simulink model "line_buffer_11x11"  (R2015a)
settings: Solver=ode45  StartTime=0.0  StopTime=10.0  RelTol=1e-3
InitFcn:
  | %% DSPBuilder Start
  | alt_dspbuilder_update_model(bdroot)
  | %% DSPBuilder End
libraries: allblocks_alteradspbuilder2 x11
settings Model: Creator=ASUS  LastModifiedBy=ASUS

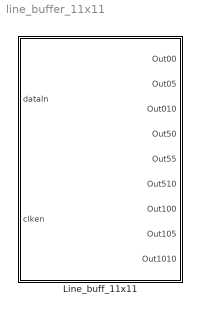
== system line_buffer_11x11 ==
  Line_buff_11x11 : Subsystem

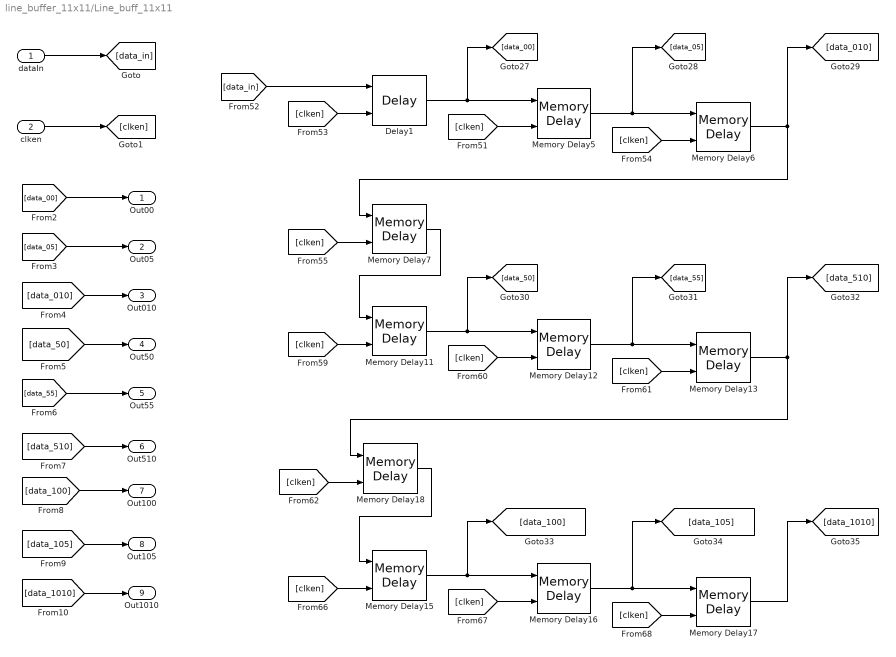
== system line_buffer_11x11/Line_buff_11x11 ==
  dataIn : Inport
  clken : Inport  Port=2
  Delay1 : allblocks_alteradspbuilder2/Delay  pipeline=1  pipeline_display=1  ClockPhase=1  use_ena=on  use_sclr=off  allowFloatingPointOverride=on  logOutputs=off  logFile=C:\Users\ASUS\Desktop\sift_fpga_final\Octave_1\line_buffer\tb_line_buffer_15x15\line%5Fbuffer%5F15x15_Line%5Fbuff%5F11x11_Delay1.fixedpointlog  use_init=off  reset_value=1
  Memory Delay11 : allblocks_alteradspbuilder2/Memory Delay  BusType=Unsigned Integer  bwl=8  bwr=0  pipeline=630  pipeline_display=630  ram_type=AUTO  use_ena=on  use_sclr=off  allowFloatingPointOverride=on  logOutputs=off  logFile=C:\Users\ASUS\Desktop\sift_fpga_final\Octave_1\line_buffer\tb_line_buffer_15x15\line%5Fbuffer%5F15x15_Line%5Fbuff%5F11x11_Memory+Delay11.fixedpointlog
  Memory Delay12 : allblocks_alteradspbuilder2/Memory Delay  BusType=Unsigned Integer  bwl=8  bwr=0  pipeline=5  pipeline_display=5  ram_type=AUTO  use_ena=on  use_sclr=off  allowFloatingPointOverride=on  logOutputs=off  logFile=C:\Users\ASUS\Desktop\sift_fpga_final\Octave_1\line_buffer\tb_line_buffer_15x15\line%5Fbuffer%5F15x15_Line%5Fbuff%5F11x11_Memory+Delay12.fixedpointlog
  Memory Delay13 : allblocks_alteradspbuilder2/Memory Delay  BusType=Unsigned Integer  bwl=8  bwr=0  pipeline=5  pipeline_display=5  ram_type=AUTO  use_ena=on  use_sclr=off  allowFloatingPointOverride=on  logOutputs=off  logFile=C:\Users\ASUS\Desktop\sift_fpga_final\Octave_1\line_buffer\tb_line_buffer_15x15\line%5Fbuffer%5F15x15_Line%5Fbuff%5F11x11_Memory+Delay13.fixedpointlog
  Memory Delay15 : allblocks_alteradspbuilder2/Memory Delay  BusType=Unsigned Integer  bwl=8  bwr=0  pipeline=630  pipeline_display=630  ram_type=AUTO  use_ena=on  use_sclr=off  allowFloatingPointOverride=on  logOutputs=off  logFile=C:\Users\ASUS\Desktop\sift_fpga_final\Octave_1\line_buffer\tb_line_buffer_15x15\line%5Fbuffer%5F15x15_Line%5Fbuff%5F11x11_Memory+Delay15.fixedpointlog
  Memory Delay16 : allblocks_alteradspbuilder2/Memory Delay  BusType=Unsigned Integer  bwl=8  bwr=0  pipeline=5  pipeline_display=5  ram_type=AUTO  use_ena=on  use_sclr=off  allowFloatingPointOverride=on  logOutputs=off  logFile=C:\Users\ASUS\Desktop\sift_fpga_final\Octave_1\line_buffer\tb_line_buffer_15x15\line%5Fbuffer%5F15x15_Line%5Fbuff%5F11x11_Memory+Delay16.fixedpointlog
  Memory Delay17 : allblocks_alteradspbuilder2/Memory Delay  BusType=Unsigned Integer  bwl=8  bwr=0  pipeline=5  pipeline_display=5  ram_type=AUTO  use_ena=on  use_sclr=off  allowFloatingPointOverride=on  logOutputs=off  logFile=C:\Users\ASUS\Desktop\sift_fpga_final\Octave_1\line_buffer\tb_line_buffer_15x15\line%5Fbuffer%5F15x15_Line%5Fbuff%5F11x11_Memory+Delay17.fixedpointlog
  Memory Delay18 : allblocks_alteradspbuilder2/Memory Delay  BusType=Unsigned Integer  bwl=8  bwr=0  pipeline=640*4  pipeline_display=2560  ram_type=AUTO  use_ena=on  use_sclr=off  allowFloatingPointOverride=on  logOutputs=off  logFile=C:\Users\ASUS\Desktop\sift_fpga_final\Octave_1\line_buffer\tb_line_buffer_15x15\line%5Fbuffer%5F15x15_Line%5Fbuff%5F11x11_Memory+Delay18.fixedpointlog
  Memory Delay5 : allblocks_alteradspbuilder2/Memory Delay  BusType=Unsigned Integer  bwl=8  bwr=0  pipeline=5  pipeline_display=5  ram_type=AUTO  use_ena=on  use_sclr=off  allowFloatingPointOverride=on  logOutputs=off  logFile=C:\Users\ASUS\Desktop\sift_fpga_final\Octave_1\line_buffer\tb_line_buffer_15x15\line%5Fbuffer%5F15x15_Line%5Fbuff%5F11x11_Memory+Delay5.fixedpointlog
  Memory Delay6 : allblocks_alteradspbuilder2/Memory Delay  BusType=Unsigned Integer  bwl=8  bwr=0  pipeline=5  pipeline_display=5  ram_type=AUTO  use_ena=on  use_sclr=off  allowFloatingPointOverride=on  logOutputs=off  logFile=C:\Users\ASUS\Desktop\sift_fpga_final\Octave_1\line_buffer\tb_line_buffer_15x15\line%5Fbuffer%5F15x15_Line%5Fbuff%5F11x11_Memory+Delay6.fixedpointlog
  Memory Delay7 : allblocks_alteradspbuilder2/Memory Delay  BusType=Unsigned Integer  bwl=8  bwr=0  pipeline=640*4  pipeline_display=2560  ram_type=AUTO  use_ena=on  use_sclr=off  allowFloatingPointOverride=on  logOutputs=off  logFile=C:\Users\ASUS\Desktop\sift_fpga_final\Octave_1\line_buffer\tb_line_buffer_15x15\line%5Fbuffer%5F15x15_Line%5Fbuff%5F11x11_Memory+Delay7.fixedpointlog
  Out00 : Outport
  Out05 : Outport  Port=2
  Out010 : Outport  Port=3
  Out50 : Outport  Port=4
  Out55 : Outport  Port=5
  Out510 : Outport  Port=6
  Out100 : Outport  Port=7
  Out105 : Outport  Port=8
  Out1010 : Outport  Port=9
  wires:
  [clken] -> Memory Delay11/2
  [clken] -> Memory Delay17/2
  [clken] -> Memory Delay6/2
  Memory Delay6/1 -> [data_010], Memory Delay7/1
  [clken] -> Memory Delay18/2
  Memory Delay18/1 -> Memory Delay15/1
  Memory Delay13/1 -> Memory Delay18/1, [data_510]
  [clken] -> Memory Delay15/2
  [clken] -> Memory Delay16/2
  Memory Delay17/1 -> [data_1010]
  Memory Delay16/1 -> Memory Delay17/1, [data_105]
  Memory Delay15/1 -> Memory Delay16/1, [data_100]
  [clken] -> Memory Delay7/2
  [clken] -> Memory Delay12/2
  Memory Delay11/1 -> Memory Delay12/1, [data_50]
  Memory Delay12/1 -> Memory Delay13/1, [data_55]
  Memory Delay7/1 -> Memory Delay11/1
  [clken] -> Memory Delay13/2
  [data_55] -> Out55/1
  [data_010] -> Out010/1
  [data_05] -> Out05/1
  clken/1 -> [clken]
  [data_00] -> Out00/1
  [data_50] -> Out50/1
  [data_100] -> Out100/1
  [data_510] -> Out510/1
  [data_1010] -> Out1010/1
  dataIn/1 -> [data_in]
  [data_105] -> Out105/1
  [clken] -> Memory Delay5/2
  Delay1/1 -> Memory Delay5/1, [data_00]
  [clken] -> Delay1/2
  [data_in] -> Delay1/1
  Memory Delay5/1 -> Memory Delay6/1, [data_05]
